simulink model "Damping_Parameter_draft"  (Simulink 7.5)
settings: Solver=ode45  StartTime=0.0  StopTime=10.0  RelTol=1e-3
libraries: dspmtrx3 x5, dspinverses x1
settings Model: Creator=konstantinos  LastModifiedBy=konstantinos

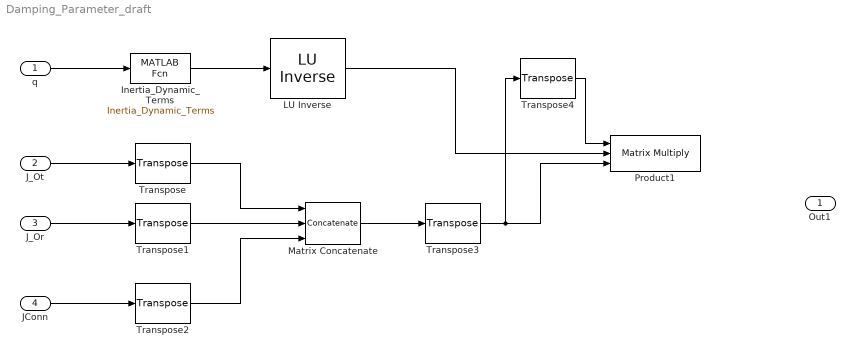
== system Damping_Parameter_draft ==
  q : Inport  OutDataType=fixdt(1, 16)  OutScaling=2^0
  J_Ot : Inport  Port=2  OutDataType=fixdt(1, 16)  OutScaling=2^0
  J_Or : Inport  Port=3  OutDataType=fixdt(1, 16)  OutScaling=2^0
  JConn : Inport  Port=4  OutDataType=fixdt(1, 16)  OutScaling=2^0
  " LU Inverse" : dspinverses/ LU Inverse  SystemSampleTime=-1
  Inertia_Dynamic_Terms : MATLABFcn  MATLABFcn=Inertia_Dynamic_Terms
  Matrix Concatenate : Concatenate  NumInputs=3  Mode=Multidimensional array  ConcatenateDimension=2
  Product1 : Product  Inputs=3  Multiplication=Matrix(*)  OutDataType=fixdt(1, 16)  OutScaling=2^0  RndMeth=Zero
  Transpose{,1..4} (5 alike) : dspmtrx3/Transpose  SystemSampleTime=-1  Hermitian=off  overflowFlag=off
  Out1 : Outport  OutDataType=fixdt(1, 16)  OutScaling=2^0
  wires:
  q/1 -> Inertia_Dynamic_Terms/1
  J_Ot/1 -> Transpose/1
  J_Or/1 -> Transpose1/1
  JConn/1 -> Transpose2/1
  Transpose/1 -> Matrix Concatenate/1
  Transpose1/1 -> Matrix Concatenate/2
  Transpose2/1 -> Matrix Concatenate/3
  Matrix Concatenate/1 -> Transpose3/1
  Inertia_Dynamic_Terms/1 -> " LU Inverse"/1
  " LU Inverse"/1 -> Product1/2
  Transpose3/1 -> Product1/3, Transpose4/1
  Transpose4/1 -> Product1/1
